simulink model "ControllerPI_TestBed"  (R2012b)
settings: Solver=ode4  StartTime=0.0  StopTime=10  FixedStep=0.2  RelTol=1e-3
undefined symbols (not defined in the file): MWS
libraries: Lib_Cntrl_SimplePIcontroller_TMATS x1
settings Model: Creator=jwchapm2  LastModifiedBy=jwchapm2

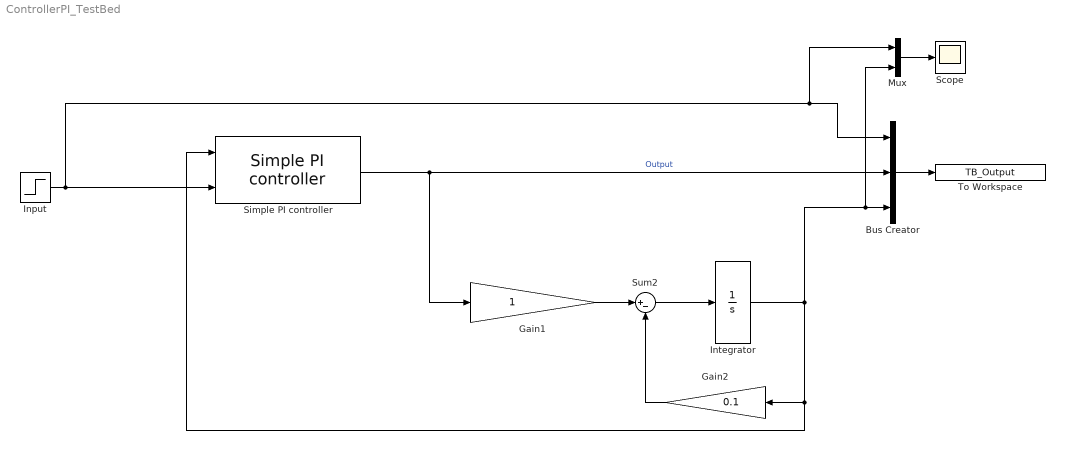
== system ControllerPI_TestBed ==
  Bus Creator : BusCreator  Inputs=3
  Gain1 : Gain
  Gain2 : Gain  Gain=0.1
  Input : Step  Time=MWS.ControllerPI.Step_Time  Before=MWS.ControllerPI.Step_IV  After=MWS.ControllerPI.Inp  SampleTime=0
  Integrator : Integrator  InitialCondition=MWS.ControllerPI.IC
  Mux : Mux  Inputs=2
  Scope : Scope
  Simple PI controller : Lib_Cntrl_SimplePIcontroller_TMATS/Simple PI controller  Kp_M=MWS.ControllerPI.Gain  Ki_M=MWS.ControllerPI.Tau  PI_IC_M=MWS.ControllerPI.IC
  Sum2 : Sum  Inputs=|+-
  To Workspace : ToWorkspace  VariableName=TB_Output  SampleTime=-1
  wires:
  Simple PI controller/1 -> Gain1/1, Bus Creator/2  "Output"
  Bus Creator/1 -> To Workspace/1
  Input/1 -> Simple PI controller/2, Mux/1, Bus Creator/1
  Gain1/1 -> Sum2/1
  Sum2/1 -> Integrator/1
  Gain2/1 -> Sum2/2
  Integrator/1 -> Mux/2, Bus Creator/3, Simple PI controller/1, Gain2/1
  Mux/1 -> Scope/1
